simulink model "sim_3"  (R2020a)
settings: Solver=FixedStepAuto  StartTime=0.0  StopTime=tf  FixedStep=0.05  RelTol=1e-3
values from neighbouring files (symbols this model uses):
  D = sqrt(4*K)    [computations_better.m]    (also in dmp.m)
  f_new = gaussian_basis(s,1,100,50,f_s)    [computations_better.m]
  g = x(length(x))    [computations_better.m]    (also in dmp.m)
  K = exp(-h.*(sn-Cs).^2)    [computations_better.m]    (also in dmp.m = 1; gaussian_basis.m)
  s = exp(-alp_s*t/tau)    [computations_better.m]    (also in dmp.m)
  tau = 1    [computations_better.m]    (also in dmp.m)
  x0 = x(1)    [computations_better.m]    (also in dmp.m)
  y = xn    [computations_better.m]    (also in forward_kin.m = [y;a1*sin(q(i,1)) + a2*sin(q(i,1)+q(i,2))]; genTraj.m = polyval(py,timeS); genTraj2.m = [])
settings Model: Creator=sirius  LastModifiedBy=sirius

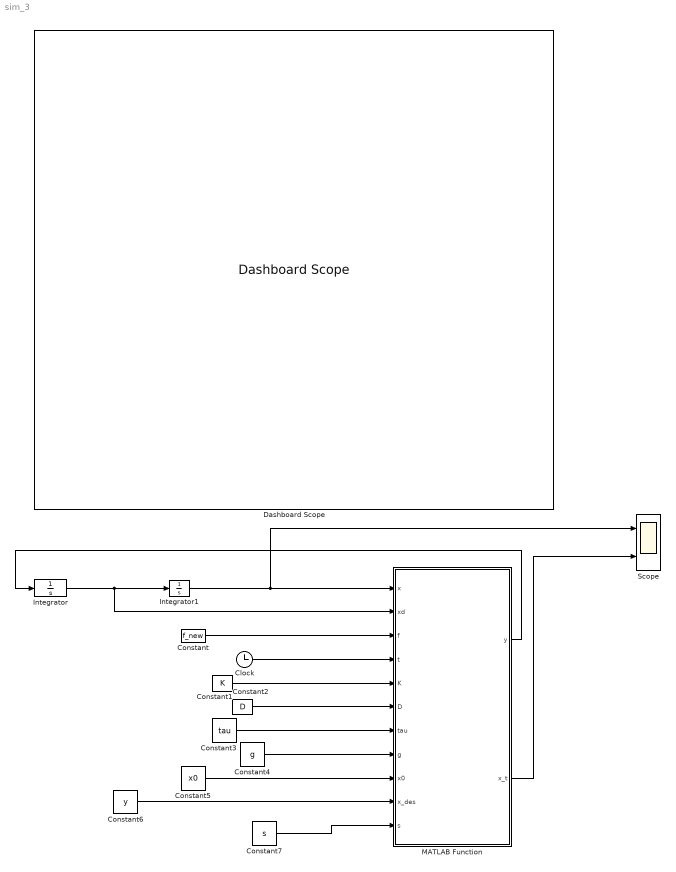
== system sim_3 ==
  Clock : Clock
  Constant : Constant  Value=f_new
  Constant1 : Constant  Value=K
  Constant2 : Constant  Value=D
  Constant3 : Constant  Value=tau
  Constant4 : Constant  Value=g
  Constant5 : Constant  Value=x0
  Constant6 : Constant  Value=y
  Constant7 : Constant  Value=s
  Dashboard Scope : DashboardScope
  Integrator : Integrator
  Integrator1 : Integrator  InitialCondition=x0
  MATLAB Function : MATLAB Function  TreatAsAtomicUnit=on
  Scope : Scope  NumInputPorts=2
  wires:
  Integrator/1 -> MATLAB Function/2(xd), Integrator1/1
  MATLAB Function/1(y) -> Integrator/1
  Constant/1 -> MATLAB Function/3(f)
  Clock/1 -> MATLAB Function/4(t)
  Integrator1/1 -> Scope/1, MATLAB Function/1(x)
  Constant1/1 -> MATLAB Function/5(K)
  Constant2/1 -> MATLAB Function/6(D)
  Constant3/1 -> MATLAB Function/7(tau)
  Constant5/1 -> MATLAB Function/9(x0)
  Constant4/1 -> MATLAB Function/8(g)
  MATLAB Function/2(x_t) -> Scope/2
  Constant6/1 -> MATLAB Function/10(x_des)
  Constant7/1 -> MATLAB Function/11(s)

== matlab function sim_3/MATLAB Function ==
  data: x input; xd input; y output; f input; t input; K input; D input; tau input; g input; x0 input; x_des input; x_t output; s input
function [y,x_t]= fcn(x, xd, f, t,K,D,tau,g,x0,x_des,s)
i = 1+ round(t/0.001);

% y = (K*(g-x) - D*tau*xd + (g-x0)*f(1+i))/(tau^2) ;

y = K*(g-x) - D*tau*xd - K*(g-x0)*s(i) + K*f(i);

x_t = x_des(i);
